simulink model "chap11_1sim"  (R2023b)
settings: Solver=ode45  StartTime=0.0  StopTime=20  RelTol=1e-3
settings Model: Creator=CorgiQvm  LastModifiedBy=CorgiQvm
settings DataIOCC: SaveFormat=Array  ReturnWorkspaceOutputs=off

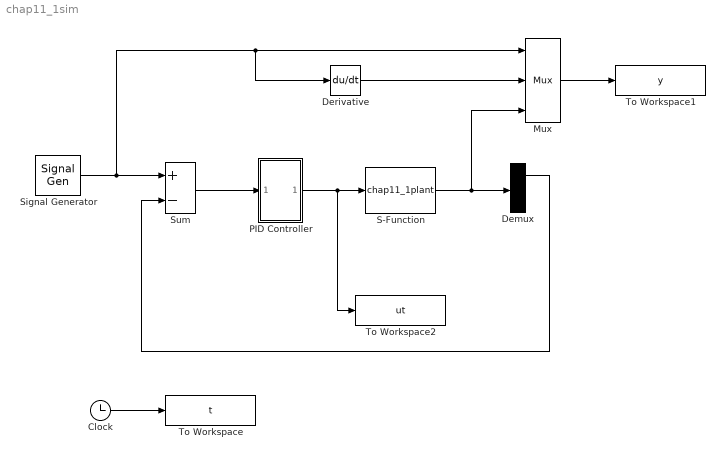
== system chap11_1sim ==
  Clock : Clock
  Demux : Demux  Outputs=2
  Derivative : Derivative
  Mux : Mux  Inputs=3
  PID Controller : Subsystem  mask{P=20, I=0, D=5}
      mask prompts: P "Proportional"; I "Integral"; D "Derivative"
      mask DialogControl ParameterGroupVar Prompt: 参数
      mask Display: disp('PID')
  S-Function : S-Function  FunctionName=chap11_1plant  SFunctionDeploymentMode=off  EnableBusSupport=off
  Signal Generator : SignalGenerator  Amplitude=0.1  Frequency=0.10
  Sum : Sum  Inputs=+-  InputSameDT=on  SaturateOnIntegerOverflow=on  OutDataTypeStr=Inherit: Same as first input
  To Workspace : ToWorkspace  VariableName=t  SampleTime=-1
  To Workspace1 : ToWorkspace  VariableName=y  SampleTime=-1
  To Workspace2 : ToWorkspace  VariableName=ut  SampleTime=-1
  wires:
  Signal Generator/1 -> Derivative/1, Mux/1, Sum/1
  Sum/1 -> PID Controller/1(In_1)
  PID Controller/1(Out1) -> To Workspace2/1, S-Function/1
  S-Function/1 -> Mux/3, Demux/1
  Demux/1 -> Sum/2
  Clock/1 -> To Workspace/1
  Derivative/1 -> Mux/2
  Mux/1 -> To Workspace1/1

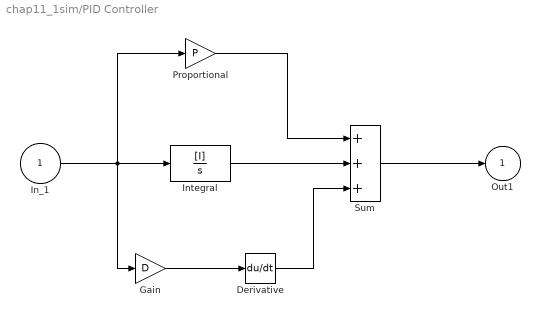
== system chap11_1sim/PID Controller ==
  In_1 : Inport
  Derivative : Derivative
  Gain : Gain  Gain=D  SaturateOnIntegerOverflow=on  OutDataTypeStr=Inherit: Same as input  ParamDataTypeStr=Inherit: Same as input
  Integral : TransferFcn  Numerator=[I]  Denominator=[1 0]
  Proportional : Gain  Gain=P  SaturateOnIntegerOverflow=on  OutDataTypeStr=Inherit: Same as input  ParamDataTypeStr=Inherit: Same as input
  Sum : Sum  Inputs=+++  InputSameDT=on  SaturateOnIntegerOverflow=on  OutDataTypeStr=Inherit: Same as first input
  Out1 : Outport
  wires:
  Derivative/1 -> Sum/3
  Proportional/1 -> Sum/1
  Sum/1 -> Out1/1
  Integral/1 -> Sum/2
  In_1/1 -> Gain/1, Proportional/1, Integral/1
  Gain/1 -> Derivative/1
